simulink model "P4p2_integral"  (R2014a)
settings: Solver=ode1  StartTime=0.0  StopTime=inf  FixedStep=0.002  RelTol=1e-3
PostLoadFcn:
  | qc_set_target_type(getConfigSet(bdroot, 'QUARC Default Target Configuration'));
values from neighbouring files (symbols this model uses):
  A_est = A_e-L*C_e    [P4p2_integral_init.m]    (also in init_heli_all.m)
  B_e = [[0  0] ... (first row only)    [P4p2_integral_init.m]    (also in init_heli_all.m = [[0 0])
  C_e = [[1 0 0 0 0 0] ... (first row only)    [P4p2_integral_init.m]    (also in init_heli_all.m)
  Joystick_gain_x = 0.8    [P4p2_integral_init.m]    (also in init_heli_all.m)
  Joystick_gain_y = -1    [P4p2_integral_init.m]    (also in init_heli_all.m)
  K = lqr(A, B, Q, R)    [P4p2_integral_init.m]    (also in init_heli_all.m)
  L = place(A_e',C_e',poles)'    [P4p2_integral_init.m]    (also in init_heli_all.m)
  P = inv(C0*inv(B0*K0-A0)*B0)    [P4p2_integral_init.m]    (also in init_heli_all.m)
  v_s_star = 6.5    [P4p2_integral_init.m]    (also in init_heli_all.m = 6.6)
undefined symbols (not defined in the file or in its folder): HIL, qc_get_step_size
libraries: simulink_extras x6, quarc_library x4
settings Model: SimulationMode=external  ExtModeTrigDuration=5000  Creator=Rchan  LastModifiedBy=henrikdf
settings SolverCC: PositivePriorityOrder=on
settings DataIOCC: SignalLoggingSaveFormat=ModelDataLogs
settings OptimizationCC: ExpressionDepthLimit=2147483647  InitFltsAndDblsToZero=on
settings DebuggingCC: SaveWithParameterizedLinksMsg=none  UnderspecifiedInitializationDetection=Classic  MultiTaskDSMMsg=warning  MultiTaskCondExecSysMsg=none  FcnCallInpInsideContextMsg=UseLocalSettings  StateNameClashWarn=warning
settings RTWCC: SystemTargetFile=quarc_win64.tlc  TemplateMakefile=quarc_default_tmf  Description=QUARC Win64 Target  ProcessScript=quarc_win64_make_rtw_hook
settings STFCustomTargetCC: CPPClassGenCompliant=on
settings GRTTargetCC: ParMdlRefBuildCompliant=off  CompOptLevelCompliant=off  CombineOutputUpdateFcns=off  MatFileLogging=off  GRTInterface=on  ExtMode=on  ExtModeMexFile=quarc_comm

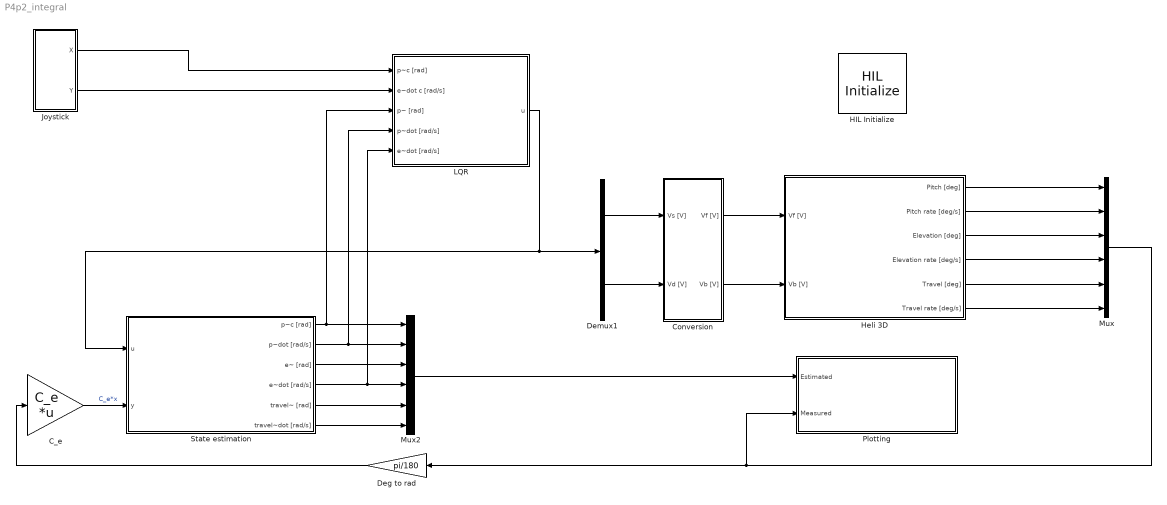
== system P4p2_integral ==
  C_e : Gain  Gain=C_e  Multiplication=Matrix(K*u)
  Conversion : Subsystem
  Deg to rad : Gain  Gain=pi/180
  Demux1 : Demux  Outputs=2
  HIL Initialize : quarc_library/Data Acquisition/Generic/Configuration/HIL Initialize  Priority=-99  object_name=HIL-1  board_type=q8_usb  board_number=0  board_options=update_rate=normal;decimation=1  exclusive=off  active=off  hardware_clocks=[0:2]  clock_modes=[]  initial_clock_frequencies=[]  set_clock_params_at_start=off  set_clock_params_at_switch_in=off  set_clock_frequencies_at_start=off  set_clock_frequencies_at_switch_in=off  analog_input_channels=[0:7]  analog_input_maximums=10  analog_input_minimums=-10  set_analog_input_params_at_start=on  set_analog_input_params_at_switch_in=off  analog_output_channels=[0:7]  analog_output_maximums=10  analog_output_minimums=-10  initial_analog_outputs=[0]  final_analog_outputs=[0]  watchdog_analog_outputs=0  set_analog_output_params_at_start=on  set_analog_output_params_at_switch_in=off  set_analog_outputs_at_start=on  set_analog_outputs_at_switch_in=off  set_analog_outputs_at_terminate=on  set_analog_outputs_at_switch_out=off  set_analog_outputs_on_watchdog=off  digital_input_channels=[]  digital_output_channels=[]  digital_output_configuration=[]  initial_digital_outputs=[1]  final_digital_outputs=[1]  watchdog_digital_outputs=[1]  set_digital_output_params_at_start=off  set_digital_output_params_at_switch_in=off  set_digital_outputs_at_start=on  set_digital_outputs_at_switch_in=off  set_digital_outputs_at_terminate=on  set_digital_outputs_at_switch_out=off  set_digital_outputs_on_watchdog=off  encoder_channels=[0:7]  quadrature=[4]  encoder_filter_frequency=[]  initial_encoder_counts=[0]  set_encoder_params_at_start=on  set_encoder_params_at_switch_in=off  set_encoder_counts_at_start=on  set_encoder_counts_at_switch_in=off  pwm_channels=[0:7]  pwm_modes=0  pwm_frequency=99.532799999999995e6/4095  pwm_configuration=[0]  pwm_alignment=[0]  pwm_polarity=[1]  pwm_leading_deadband=[0]  pwm_trailing_deadband=[0]  initial_pwm_outputs=[0]  final_pwm_outputs=[0]  watchdog_pwm_outputs=[0]  set_pwm_params_at_start=on  set_pwm_params_at_switch_in=off  set_pwm_outputs_at_start=on  set_pwm_outputs_at_switch_in=off  set_pwm_outputs_at_terminate=on  set_pwm_outputs_at_switch_out=off  set_pwm_outputs_on_watchdog=off  other_output_channels=[]  initial_other_outputs=[]  final_other_outputs=[]  watchdog_other_outputs=[]  set_other_outputs_at_start=off  set_other_outputs_at_switch_in=off  set_other_outputs_at_terminate=off  set_other_outputs_at_switch_out=off  set_other_outputs_on_watchdog=off
  Heli 3D : Subsystem
  Joystick : Subsystem
  LQR : Subsystem
  Mux : Mux  Inputs=6
  Mux2 : Mux  Inputs=6
  Plotting : Subsystem
  State estimation : Subsystem
  wires:
  Conversion/2(Vb [V]) -> Heli 3D/2(Vb [V])
  Conversion/1(Vf [V]) -> Heli 3D/1(Vf [V])
  Demux1/2 -> Conversion/2(Vd [V])
  Mux2/1 -> Plotting/1(Estimated)
  State estimation/1(p~c [rad]) -> Mux2/1, LQR/3(p~ [rad])
  State estimation/2(p~dot [rad/s]) -> LQR/4(p~dot [rad/s]), Mux2/2
  State estimation/3(e~ [rad]) -> Mux2/3
  State estimation/5(travel~ [rad]) -> Mux2/5
  State estimation/6(travel~dot [rad/s]) -> Mux2/6
  Heli 3D/1(Pitch [deg]) -> Mux/1
  Heli 3D/2(Pitch rate [deg/s]) -> Mux/2
  Heli 3D/3(Elevation [deg]) -> Mux/3
  Heli 3D/4(Elevation rate [deg/s]) -> Mux/4
  Heli 3D/5(Travel [deg]) -> Mux/5
  Heli 3D/6(Travel rate [deg/s]) -> Mux/6
  State estimation/4(e~dot [rad/s]) -> LQR/5(e~dot [rad/s]), Mux2/4
  LQR/1(u) -> State estimation/1(u), Demux1/1
  Joystick/1(X) -> LQR/1(p~c [rad])
  Joystick/2(Y) -> LQR/2(e~dot c [rad/s])
  Demux1/1 -> Conversion/1(Vs [V])
  Deg to rad/1 -> C_e/1
  C_e/1 -> State estimation/2(y)  "C_e*x"
  Mux/1 -> Plotting/2(Measured), Deg to rad/1

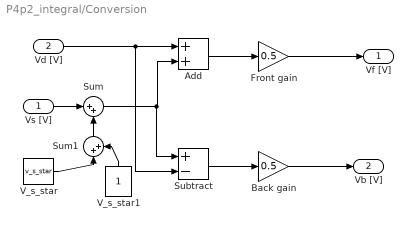
== system P4p2_integral/Conversion ==
  Vs [V] : Inport
  Vd [V] : Inport  Port=2
  Add : Sum
  Back gain : Gain  Gain=0.5
  Front gain : Gain  Gain=0.5
  Subtract : Sum  Inputs=+-
  Sum : Sum  Inputs=|++
  Sum1 : Sum  Inputs=|++
  V_s_star : Constant  Value=v_s_star
  V_s_star1 : Constant
  Vf [V] : Outport
  Vb [V] : Outport  Port=2
  wires:
  Vd [V]/1 -> Subtract/2, Add/1
  Subtract/1 -> Back gain/1
  Back gain/1 -> Vb [V]/1
  Add/1 -> Front gain/1
  Front gain/1 -> Vf [V]/1
  Vs [V]/1 -> Sum/1
  Sum/1 -> Subtract/1, Add/2
  V_s_star/1 -> Sum1/1
  Sum1/1 -> Sum/2
  V_s_star1/1 -> Sum1/2

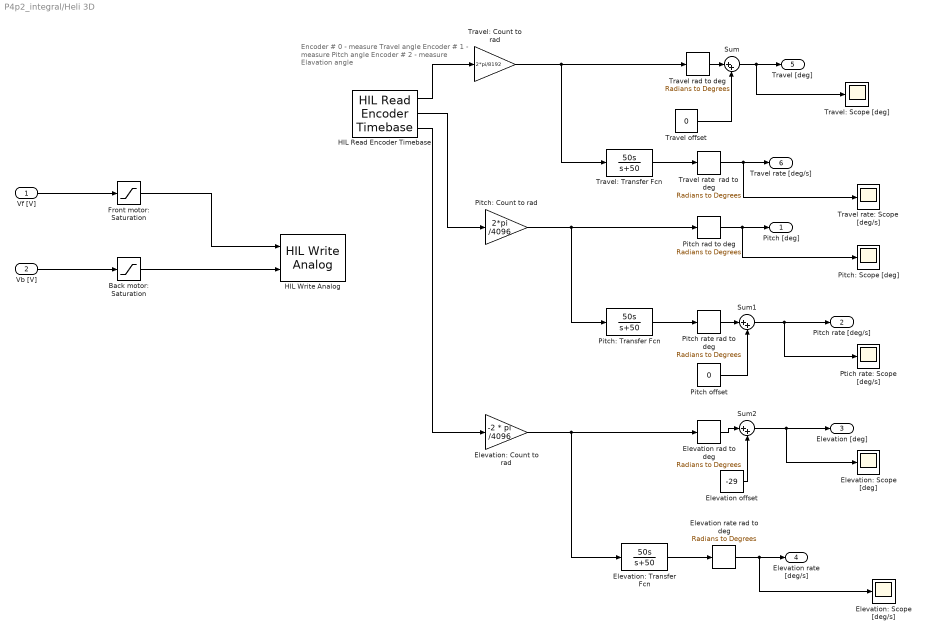
== system P4p2_integral/Heli 3D ==
  note: Encoder # 0 - measure Travel angle
      | Encoder # 1 - measure Pitch angle
      | Encoder # 2 - measure Elavation angle
  Vf [V] : Inport
  Vb [V] : Inport  Port=2
  Back motor: Saturation : Saturate  UpperLimit=5  LowerLimit=-5
  Elevation offset : Constant  Value=-29
  Elevation rad to deg : simulink_extras/Transformations/Radians to Degrees
  Elevation rate rad to deg : simulink_extras/Transformations/Radians to Degrees
  Elevation: Count to rad : Gain  Gain=-2 * pi /4096
  Elevation: Scope [deg/s] : Scope
      settings: YMin=-15  YMax=15  SaveName=ScopeData13
  Elevation: Scope [deg] : Scope
      settings: TimeRange=10  YMin=-30  YMax=10  SaveName=ScopeData12
  Elevation: Transfer Fcn : TransferFcn  Numerator=[50 0]  Denominator=[1 50]
  Front motor: Saturation : Saturate  UpperLimit=5  LowerLimit=-5
  HIL Read Encoder Timebase : quarc_library/Data Acquisition/Generic/Timebases/HIL Read Encoder Timebase  object_name=HIL-1  clock=0  channels=[0:2]  samples_in_buffer=max(ceil(1/qc_get_step_size), 1)  active=on  vector_output=off  data_type_mode=Inherit via back propagation  data_type=double
  HIL Write Analog : quarc_library/Data Acquisition/Generic/Immediate I//O/HIL Write Analog  object_name=HIL-1  channels=[0:1]  sample_time=-1  active=off  vector_input=off
  "Pitch offset " : Constant  Value=0
  Pitch rad to deg : simulink_extras/Transformations/Radians to Degrees
  Pitch rate rad to deg : simulink_extras/Transformations/Radians to Degrees
  Pitch: Count to rad : Gain  Gain=2*pi /4096
  Pitch: Scope [deg] : Scope
      settings: YMin=-15  YMax=15  SaveName=ScopeData10
  Pitch: Transfer Fcn : TransferFcn  Numerator=[50 0]  Denominator=[1 50]
  Ptich rate: Scope [deg/s] : Scope
      settings: YMin=-15  YMax=15  SaveName=ScopeData11
  Sum : Sum  Inputs=|++
  Sum1 : Sum  Inputs=|++
  Sum2 : Sum  Inputs=|++
  "Travel offset " : Constant  Value=0
  Travel rad to deg : simulink_extras/Transformations/Radians to Degrees
  Travel rate  rad to deg : simulink_extras/Transformations/Radians to Degrees
  Travel rate: Scope [deg/s] : Scope
      settings: YMin=-15  YMax=15  SaveName=ScopeData9
  Travel: Count to rad : Gain  Gain=2*pi/8192
  Travel: Scope [deg] : Scope
      settings: YMin=-15  YMax=15  SaveName=ScopeData8
  Travel: Transfer Fcn : TransferFcn  Numerator=[50 0]  Denominator=[1 50]
  Pitch [deg] : Outport
  Pitch rate [deg/s] : Outport  Port=2
  Elevation [deg] : Outport  Port=3
  Elevation rate [deg/s] : Outport  Port=4
  Travel [deg] : Outport  Port=5
  Travel rate [deg/s] : Outport  Port=6
  wires:
  HIL Read Encoder Timebase/1 -> Travel: Count to rad/1
  HIL Read Encoder Timebase/2 -> Pitch: Count to rad/1
  HIL Read Encoder Timebase/3 -> Elevation: Count to rad/1
  Travel: Count to rad/1 -> Travel: Transfer Fcn/1, Travel rad to deg/1
  Travel: Transfer Fcn/1 -> Travel rate  rad to deg/1
  Pitch: Count to rad/1 -> Pitch: Transfer Fcn/1, Pitch rad to deg/1
  Pitch: Transfer Fcn/1 -> Pitch rate rad to deg/1
  Elevation: Count to rad/1 -> Elevation: Transfer Fcn/1, Elevation rad to deg/1
  Elevation: Transfer Fcn/1 -> Elevation rate rad to deg/1
  Travel rate  rad to deg/1 -> Travel rate: Scope [deg/s]/1, Travel rate [deg/s]/1
  Pitch rad to deg/1 -> Pitch: Scope [deg]/1, Pitch [deg]/1
  Elevation rate rad to deg/1 -> Elevation: Scope [deg/s]/1, Elevation rate [deg/s]/1
  Vf [V]/1 -> Front motor: Saturation/1
  Vb [V]/1 -> Back motor: Saturation/1
  Front motor: Saturation/1 -> HIL Write Analog/1
  Back motor: Saturation/1 -> HIL Write Analog/2
  Sum/1 -> Travel: Scope [deg]/1, Travel [deg]/1
  Travel rad to deg/1 -> Sum/1
  "Travel offset "/1 -> Sum/2
  Pitch rate rad to deg/1 -> Sum1/1
  Sum1/1 -> Ptich rate: Scope [deg/s]/1, Pitch rate [deg/s]/1
  "Pitch offset "/1 -> Sum1/2
  Elevation rad to deg/1 -> Sum2/1
  Sum2/1 -> Elevation: Scope [deg]/1, Elevation [deg]/1
  Elevation offset/1 -> Sum2/2

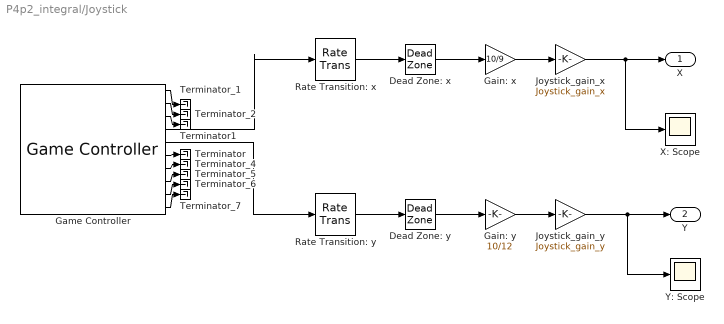
== system P4p2_integral/Joystick ==
  Dead Zone: x : DeadZone  LowerValue=-0.1  UpperValue=0.1  SaturateOnIntegerOverflow=on
  Dead Zone: y : DeadZone  LowerValue=-0.1  UpperValue=0.1  SaturateOnIntegerOverflow=on
  Gain: x : Gain  Gain=10/9
  Gain: y : Gain  Gain=10/12
  Game Controller : quarc_library/Devices/Peripherals/Target/Game Controller  controller=1  buffer_size=12  deadzone=[]  saturation=[]  sample_time=max(qc_get_step_size, 0.01)  auto_center=off  enabled=on
  Joystick_gain_x : Gain  Gain=Joystick_gain_x
  Joystick_gain_y : Gain  Gain=Joystick_gain_y
  Rate Transition: x : RateTransition
  Rate Transition: y : RateTransition
  Terminator : Terminator
  Terminator1 : Terminator
  Terminator_{1..2,4..7} (6 alike) : Terminator
  X: Scope : Scope
      settings: YMin=-1  YMax=1  SaveName=ScopeData7
  Y: Scope : Scope
      settings: YMin=-9  YMax=8  SaveName=ScopeData5
  X : Outport
  Y : Outport  Port=2
  wires:
  Rate Transition: y/1 -> Dead Zone: y/1
  Rate Transition: x/1 -> Dead Zone: x/1
  Game Controller/5 -> Rate Transition: y/1
  Game Controller/4 -> Rate Transition: x/1
  Game Controller/1 -> Terminator_1/1
  Game Controller/2 -> Terminator_2/1
  Game Controller/7 -> Terminator_4/1
  Game Controller/8 -> Terminator_5/1
  Game Controller/9 -> Terminator_6/1
  Game Controller/10 -> Terminator_7/1
  Game Controller/3 -> Terminator1/1
  Game Controller/6 -> Terminator/1
  Dead Zone: x/1 -> Gain: x/1
  Dead Zone: y/1 -> Gain: y/1
  Gain: x/1 -> Joystick_gain_x/1
  Gain: y/1 -> Joystick_gain_y/1
  Joystick_gain_x/1 -> X/1, X: Scope/1
  Joystick_gain_y/1 -> Y: Scope/1, Y/1

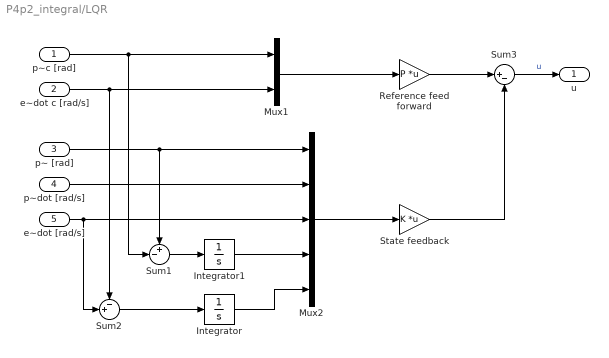
== system P4p2_integral/LQR ==
  p~c [rad] : Inport
  e~dot c [rad/s] : Inport  Port=2
  p~ [rad] : Inport  Port=3
  p~dot [rad/s] : Inport  Port=4
  e~dot [rad/s] : Inport  Port=5
  Integrator : Integrator
  Integrator1 : Integrator
  Mux1 : Mux  Inputs=2
  Mux2 : Mux  Inputs=5
  "Reference feed forward " : Gain  Gain=P  Multiplication=Matrix(K*u)
  State feedback : Gain  Gain=K  Multiplication=Matrix(K*u)
  Sum1 : Sum  Inputs=+-|
  Sum2 : Sum  Inputs=-+|
  Sum3 : Sum  Inputs=|+-
  u : Outport
  wires:
  State feedback/1 -> Sum3/2
  "Reference feed forward "/1 -> Sum3/1
  Mux2/1 -> State feedback/1
  Mux1/1 -> "Reference feed forward "/1
  Sum3/1 -> u/1  "u"
  p~ [rad]/1 -> Sum1/1, Mux2/1
  e~dot [rad/s]/1 -> Sum2/2, Mux2/3
  p~dot [rad/s]/1 -> Mux2/2
  e~dot c [rad/s]/1 -> Mux1/2, Sum2/1
  p~c [rad]/1 -> Mux1/1, Sum1/2
  Sum2/1 -> Integrator/1
  Sum1/1 -> Integrator1/1
  Integrator1/1 -> Mux2/4
  Integrator/1 -> Mux2/5

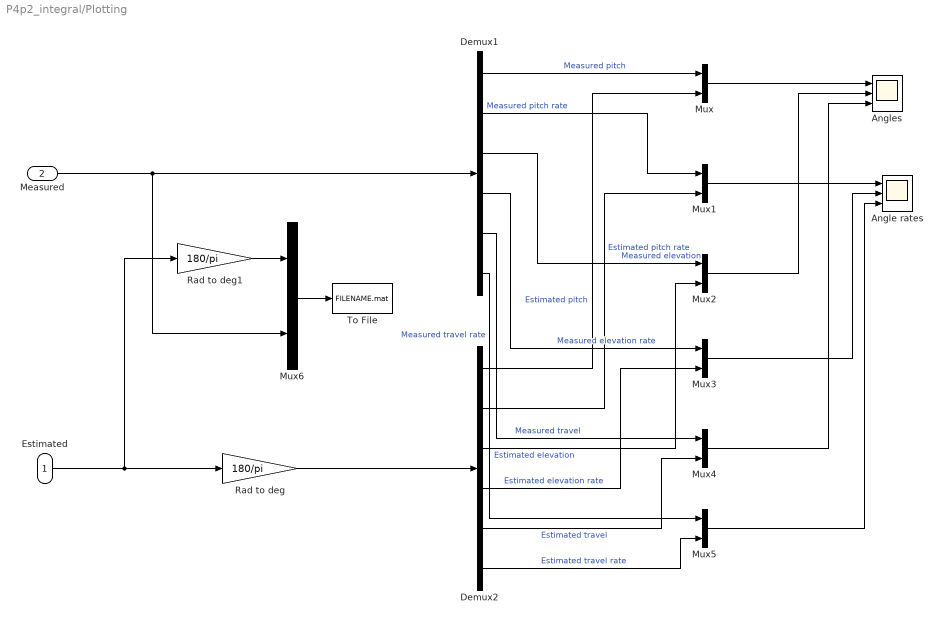
== system P4p2_integral/Plotting ==
  Estimated : Inport
  Measured : Inport  Port=2
  Angle rates : Scope  NumInputPorts=3
      settings: ShowLegends=on  TimeRange=10  YMin=-8~-4.5~59  YMax=8~4.5~65.5  SaveName=ScopeData3
  Angles : Scope  NumInputPorts=3
      settings: ShowLegends=on  TimeRange=30  YMin=-1~5.175~2325  YMax=2~5.475~2625
  Demux1 : Demux  Outputs=6
  Demux2 : Demux  Outputs=6
  Mux{,1..6} (7 alike) : Mux  Inputs=2
  Rad to deg : Gain  Gain=180/pi
  Rad to deg1 : Gain  Gain=180/pi
  To File : ToFile  Filename=FILENAME.mat
  wires:
  Mux/1 -> Angles/1
  Mux2/1 -> Angles/2
  Estimated/1 -> Rad to deg1/1, Rad to deg/1
  Demux1/1 -> Mux/1  "Measured pitch"
  Demux2/1 -> Mux/2  "Estimated pitch"
  Mux1/1 -> Angle rates/1
  Demux1/2 -> Mux1/1  "Measured pitch rate"
  Demux2/2 -> Mux1/2  "Estimated pitch rate"
  Demux1/3 -> Mux2/1  "Measured elevation"
  Demux2/3 -> Mux2/2  "Estimated elevation"
  Mux3/1 -> Angle rates/2
  Demux1/4 -> Mux3/1  "Measured elevation rate"
  Demux2/4 -> Mux3/2  "Estimated elevation rate"
  Mux4/1 -> Angles/3
  Mux5/1 -> Angle rates/3
  Demux1/5 -> Mux4/1  "Measured travel"
  Demux2/5 -> Mux4/2  "Estimated travel"
  Demux1/6 -> Mux5/1  "Measured travel rate"
  Demux2/6 -> Mux5/2  "Estimated travel rate"
  Rad to deg/1 -> Demux2/1
  Mux6/1 -> To File/1
  Measured/1 -> Mux6/2, Demux1/1
  Rad to deg1/1 -> Mux6/1

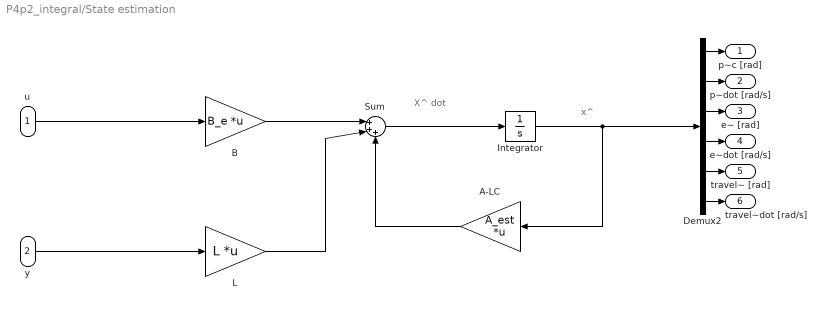
== system P4p2_integral/State estimation ==
  note: x^
  note: X^ dot
  u : Inport
  y : Inport  Port=2
  A-LC : Gain  Gain=A_est  Multiplication=Matrix(K*u)
  B : Gain  Gain=B_e  Multiplication=Matrix(K*u)
  Demux2 : Demux  Outputs=6
  Integrator : Integrator
  L : Gain  Gain=L  Multiplication=Matrix(K*u)
  Sum : Sum  Inputs=|+++
  p~c [rad] : Outport
  p~dot [rad/s] : Outport  Port=2
  e~ [rad] : Outport  Port=3
  e~dot [rad/s] : Outport  Port=4
  travel~ [rad] : Outport  Port=5
  travel~dot [rad/s] : Outport  Port=6
  wires:
  B/1 -> Sum/1
  Sum/1 -> Integrator/1
  Integrator/1 -> A-LC/1, Demux2/1
  L/1 -> Sum/2
  A-LC/1 -> Sum/3
  Demux2/2 -> p~dot [rad/s]/1
  Demux2/3 -> e~ [rad]/1
  Demux2/4 -> e~dot [rad/s]/1
  Demux2/5 -> travel~ [rad]/1
  Demux2/1 -> p~c [rad]/1
  u/1 -> B/1
  Demux2/6 -> travel~dot [rad/s]/1
  y/1 -> L/1
